simulink model "gfsk_final"  (R2022b)
settings: Solver=VariableStepAuto  StartTime=0.0  StopTime=0.1  RelTol=1e-3
undefined symbols (not defined in the file): DiscIntNeverNeededParam, j
libraries: commdigbbndpm3 x3, simulink x3, commchan3 x1, commrandsrc3 x1, commsink2 x1, phaseddetectlib x1, commsync2 x1
settings Model: Creator=Leoni Gabriel  LastModifiedBy=Leoni Gabriel

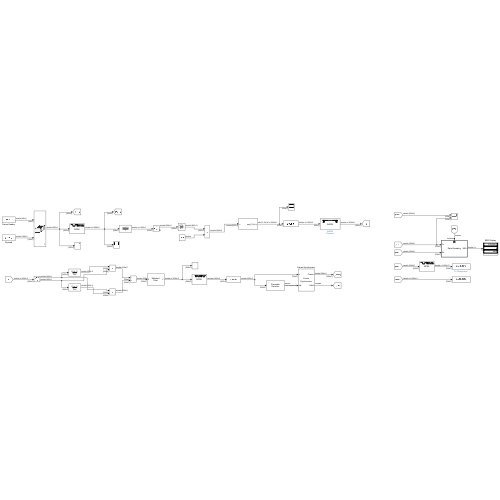
[thumbnail: Simulink's stored preview of the top-level diagram]
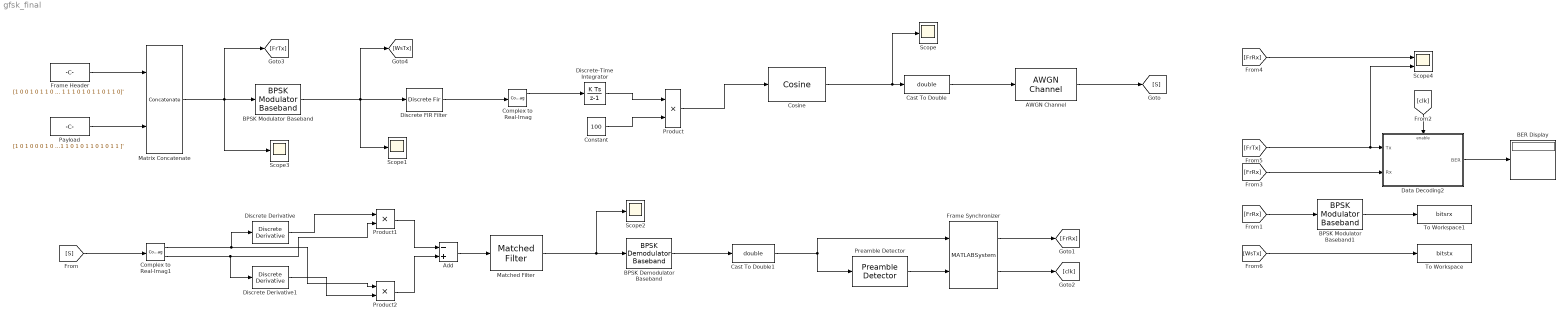
== system gfsk_final ==
  AWGN Channel : commchan3/AWGN Channel  InputProcessing=Columns as channels (frame based)  seed=67  noiseMode="Signal to noise ratio  (SNR)"  EbNodB=10  EsNodB=10  SNRdB=10  bitsPerSym=1  Ps=1  Tsym=1  variance=1
  Add : Sum  Inputs=-+  OutDataTypeStr=double
  BER Display : Display
  BPSK Demodulator Baseband : commdigbbndpm3/BPSK Demodulator Baseband  DecType=Hard decision  VarSource=Dialog  Variance=1  Ph=0  outDtype=boolean  derotateFactorWordLen=16  derotateFactorDataTypeStr=Inherit: Same word length as input  derotateFactorLastDataTypeStr=Inherit: Same word length as input
  BPSK Modulator Baseband : commdigbbndpm3/BPSK Modulator Baseband  Ph=0  outDtype=double  outWordLen=16  outUDDataType=sfix(16)  outFracLenMode=Best precision  outFracLen=15  outDataTypeStr=double  outLastDataTypeStr=double
  BPSK Modulator Baseband1 : commdigbbndpm3/BPSK Modulator Baseband  Ph=0  outDtype=double  outWordLen=16  outUDDataType=sfix(16)  outFracLenMode=Best precision  outFracLen=15  outDataTypeStr=double  outLastDataTypeStr=double
  Cast To Double : DataTypeConversion  OutDataTypeStr=double  SaturateOnIntegerOverflow=off  RndMeth=Floor
  Cast To Double1 : DataTypeConversion  OutDataTypeStr=double  SaturateOnIntegerOverflow=off  RndMeth=Floor
  Complex to Real-Imag : ComplexToRealImag
  Complex to Real-Imag1 : ComplexToRealImag
  Constant : Constant  Value=100
  Cosine : simulink/Lookup Tables/Cosine  Formula=exp(j*2*pi*u)  NumDataPoints=(2^5)+1  OutputWordLength=16  InternalRulePriority=Speed
  Data Decoding2 : Subsystem
      mask Display: disp('Data Decoding');
  Discrete Derivative : simulink/Discrete/Discrete Derivative  gainval=1.0  ICPrevScaledInput=0.0  OutMin=[]  OutMax=[]  OutDataType=fixdt(1, 16)  OutScaling=2^-10  DoSatur=off
  Discrete Derivative1 : simulink/Discrete/Discrete Derivative  gainval=1.0  ICPrevScaledInput=0.0  OutMin=[]  OutMax=[]  OutDataType=fixdt(1, 16)  OutScaling=2^-10  DoSatur=off
  Discrete FIR Filter : DiscreteFir  Coefficients="[0.0668    0.8664    0.0668]"
  Discrete-Time Integrator : DiscreteIntegrator  SampleTime=-1  ICPrevOutput=DiscIntNeverNeededParam  ICPrevScaledInput=DiscIntNeverNeededParam
  Frame Header : Constant  Value=[1 0 0 1 0 1 1 0 1 1 1 0 1 0 1 1 0 1 1 0 1 0 0 1 0 1 1 0 1 1 1 0 1 0 1 1 0 1 1 0]'  VectorParams1D=off  OutDataTypeStr=double
  Frame Synchronizer : MATLABSystem  System=comm.internal.examples.FrameSynchronizer  Input=Bit  OutputFrameLength=200  PreambleLength=40  SimulateUsing=Code generation
      mask Type: comm.internal.examples.FrameSynchronizer
      mask Display:
      | disp(['Frame' char(10) 'Synchronizer']);
      | port_label('input',1,'u');
      | port_label('input',2,'idx');
      | port_label('output',1,'Frame');
      | port_label('output',2,'Valid');
  Matched Filter : phaseddetectlib/Matched Filter  CoefficientsSource=Property  Coefficients="[0.0668    0.8664    0.0668]"  SpectrumWindow=None  CustomSpectrumWindow=@hamming  SpectrumRange=[ 0, 1e5 ]  SampleRateFromInputCheckbox=on  SampleRate=1e6  SidelobeAttenuation=30  Beta=0.5  Nbar=4  GainOutputPort=off  MaximumNumInputSamplesSource=Auto  MaximumNumInputSamples=100  SimulateUsing=Interpreted execution
  Matrix Concatenate : Concatenate  Mode=Multidimensional array
  Payload : Constant  Value=[1 0 1 0 0 0 1 0 0 1 0 1 0 1 0 1 0 0 1 1 0 1 1 0 1 0 1 0 1 1 0 1 0 1 1 0 0 1 0 0 1 0 1 1 0 1 1 1 0 1 0 1 1 0 1 1 0 1 0 0 1 0 1 1 0 1 1 1 0 1 1 0 1 0 1 1 0 1 1 1 0 1 0 0 0 1 0 0 1 0 1 0 1 0 1 0 0 1 1 0 1 1 0 1 0 1 0 1 1 0 1 0 1 1 0 0 1 0 0 1 0 1 1 0 1 1 1 0 1 0 1 1 0 1 1 0 1 0 0 1 0 1 1 0 1 1 1 0 1 1 0 1 0 1 1 0 1 0 1 1 ]'  VectorParams1D=off  OutDataTypeStr=double
  Preamble Detector : commsync2/Preamble Detector  Input=Bit  Preamble=[1 0 0 1 0 1 1 0 1 1 1 0 1 0 1 1 0 1 1 0 1 0 0 1 0 1 1 0 1 1 1 0 1 0 1 1 0 1 1 0]'  Threshold=3  DetectionMetricOutput=off  Detections=First  SimulateUsing=Code generation
  Product : Product
  Product1 : Product
  Product2 : Product
  Scope{,1..3} (4 alike) : Scope
  Scope4 : Scope  NumInputPorts=2
  To Workspace : ToWorkspace  VariableName=bitstx  SaveFormat=Timeseries  SampleTime=-1
  To Workspace1 : ToWorkspace  VariableName=bitsrx  SaveFormat=Timeseries  SampleTime=-1
  wires:
  Discrete Derivative1/1 -> Product2/2
  Product2/1 -> Add/2
  Payload/1 -> Matrix Concatenate/2
  Frame Header/1 -> Matrix Concatenate/1
  Discrete FIR Filter/1 -> Complex to Real-Imag/1
  Cast To Double1/1 -> Preamble Detector/1, Frame Synchronizer/1
  Data Decoding2/1(BER) -> BER Display/1
  Complex to Real-Imag1/2 -> Discrete Derivative1/1, Product1/2
  Complex to Real-Imag1/1 -> Discrete Derivative/1, Product2/1
  Preamble Detector/1 -> Frame Synchronizer/2
  Cosine/1 -> Cast To Double/1, Scope/1
  Matched Filter/1 -> Scope2/1, BPSK Demodulator Baseband/1
  Discrete Derivative/1 -> Product1/1
  Product1/1 -> Add/1
  BPSK Modulator Baseband1/1 -> To Workspace1/1
  Discrete-Time Integrator/1 -> Product/1
  [FrTx] -> Data Decoding2/1(Tx), Scope4/2
  BPSK Demodulator Baseband/1 -> Cast To Double1/1
  BPSK Modulator Baseband/1 -> [WsTx], Scope1/1, Discrete FIR Filter/1
  Matrix Concatenate/1 -> BPSK Modulator Baseband/1, Scope3/1, [FrTx]
  Constant/1 -> Product/2
  Product/1 -> Cosine/1
  Complex to Real-Imag/1 -> Discrete-Time Integrator/1
  [S] -> Complex to Real-Imag1/1
  Cast To Double/1 -> AWGN Channel/1
  AWGN Channel/1 -> [S]
  [clk] -> Data Decoding2/Enable
  Frame Synchronizer/2 -> [clk]
  [FrRx] -> BPSK Modulator Baseband1/1
  [FrRx] -> Data Decoding2/2(Rx)
  Frame Synchronizer/1 -> [FrRx]
  [FrRx] -> Scope4/1
  Add/1 -> Matched Filter/1
  [WsTx] -> To Workspace/1

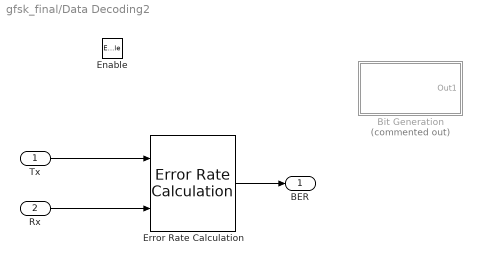
== system gfsk_final/Data Decoding2 ==
  Tx : Inport
  Rx : Inport  Port=2
  Enable : EnablePort
  Bit Generation : Subsystem  Commented=on
      mask Display: disp('Bit Frame\nGeneration')
  Error Rate Calculation : commsink2/Error Rate Calculation  N=0  st_delay=0  cp_mode=Entire frame  subframe=[]  PMode=Port  WsName=ErrorVec  RsMode2=off  stop=off  numErr=100  maxBits=1e6
  BER : Outport  VectorParamsAs1DForOutWhenUnconnected=off
  wires:
  Error Rate Calculation/1 -> BER/1
  Rx/1 -> Error Rate Calculation/2
  Tx/1 -> Error Rate Calculation/1

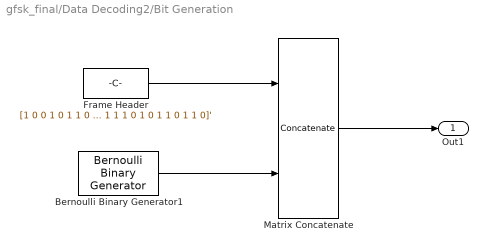
== system gfsk_final/Data Decoding2/Bit Generation ==
  Bernoulli Binary Generator1 : commrandsrc3/Bernoulli Binary Generator  ProbabilityOfZero=0.5  SeedSource=Parameter  Seed=61  SampleTime=1  SamplesPerFrame=160  OutputDataType=double  SimulateUsing=Interpreted execution
  Frame Header : Constant  Value=[1 0 0 1 0 1 1 0 1 1 1 0 1 0 1 1 0 1 1 0 1 0 0 1 0 1 1 0 1 1 1 0 1 0 1 1 0 1 1 0]'  VectorParams1D=off  OutDataTypeStr=double
  Matrix Concatenate : Concatenate  Mode=Multidimensional array
  Out1 : Outport  VectorParamsAs1DForOutWhenUnconnected=off
  wires:
  Matrix Concatenate/1 -> Out1/1
  Frame Header/1 -> Matrix Concatenate/1
  Bernoulli Binary Generator1/1 -> Matrix Concatenate/2
